simulink model "Algebric_Loops"  (R2020a)
settings: Solver=VariableStepAuto  StartTime=0.0  StopTime=10.0  RelTol=1e-3
settings Model: Creator=hussein  LastModifiedBy=hussein

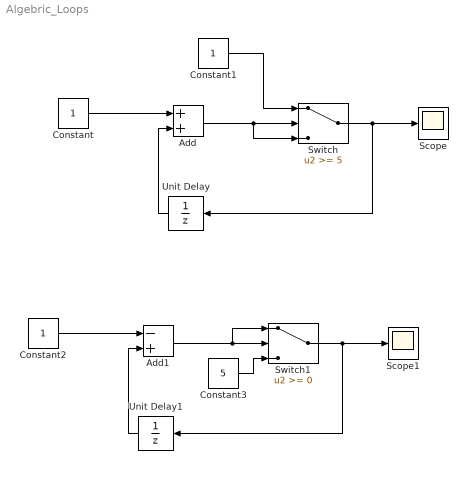
== system Algebric_Loops ==
  Add : Sum
  Add1 : Sum  Inputs=-+
  Constant : Constant
  Constant1 : Constant
  Constant2 : Constant
  Constant3 : Constant  Value=5
  Scope : Scope
  Scope1 : Scope
  Switch : Switch  Threshold=5
  Switch1 : Switch
  Unit Delay : UnitDelay  SampleTime=-1  HasFrameUpgradeWarning=on
  Unit Delay1 : UnitDelay  SampleTime=-1  HasFrameUpgradeWarning=on
  wires:
  Unit Delay/1 -> Add/2
  Constant/1 -> Add/1
  Add/1 -> Switch/3, Switch/2
  Constant1/1 -> Switch/1
  Switch/1 -> Unit Delay/1, Scope/1
  Switch1/1 -> Scope1/1, Unit Delay1/1
  Add1/1 -> Switch1/1, Switch1/2
  Constant2/1 -> Add1/1
  Unit Delay1/1 -> Add1/2
  Constant3/1 -> Switch1/3
